simulink model "Dyn_6DoF_v2_0_r2019b"  (R2022a)
settings: Solver=ode4  StartTime=0.0  StopTime=simInit.TSIM  FixedStep=simInit.dt  MaxStep=simInit.dt  RelTol=1e-3
InitFcn:
  | close all
undefined symbols (not defined in the file): act, constr, DE2019, DiscIntNeverNeededParam, ENVMT, omega_rate_max, params, simInit
libraries: simulink x14, simulink_extras x3
(part 2 of 3)

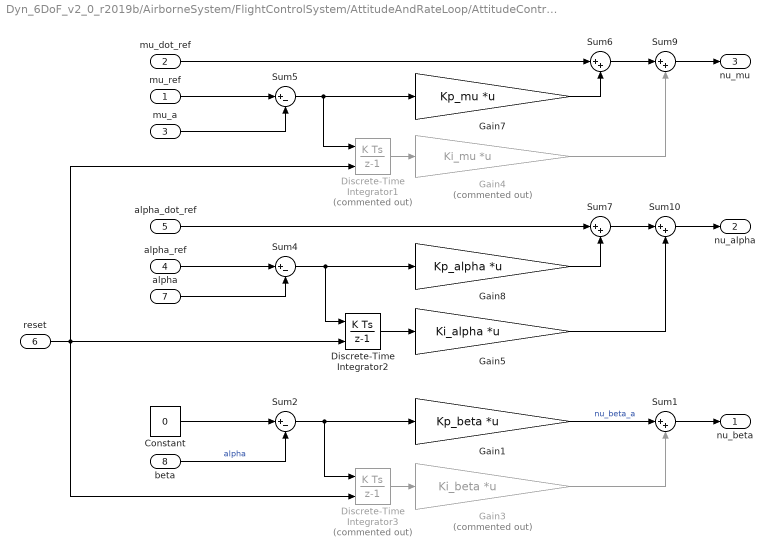
== system Dyn_6DoF_v2_0_r2019b/AirborneSystem/FlightControlSystem/AttitudeAndRateLoop/AttitudeController/PI-controller ==
  mu_ref : Inport
  mu_dot_ref : Inport  Port=2
  mu_a : Inport  Port=3
  alpha_ref : Inport  Port=4
  alpha_dot_ref : Inport  Port=5
  reset : Inport  Port=6
  alpha : Inport  Port=7
  beta : Inport  Port=8
  Constant : Constant  Value=0
  Discrete-Time Integrator1 : DiscreteIntegrator  Commented=on  ExternalReset=rising  SampleTime=-1  ICPrevOutput=DiscIntNeverNeededParam  ICPrevScaledInput=DiscIntNeverNeededParam
  Discrete-Time Integrator2 : DiscreteIntegrator  ExternalReset=either  SampleTime=-1  ICPrevOutput=DiscIntNeverNeededParam  ICPrevScaledInput=DiscIntNeverNeededParam
  Discrete-Time Integrator3 : DiscreteIntegrator  Commented=on  ExternalReset=rising  SampleTime=-1  ICPrevOutput=DiscIntNeverNeededParam  ICPrevScaledInput=DiscIntNeverNeededParam
  Gain1 : Gain  Gain=Kp_beta  Multiplication=Matrix(K*u)
  Gain3 : Gain  Commented=on  Gain=Ki_beta  Multiplication=Matrix(K*u)
  Gain4 : Gain  Commented=on  Gain=Ki_mu  Multiplication=Matrix(K*u)
  Gain5 : Gain  Gain=Ki_alpha  Multiplication=Matrix(K*u)
  Gain7 : Gain  Gain=Kp_mu  Multiplication=Matrix(K*u)
  Gain8 : Gain  Gain=Kp_alpha  Multiplication=Matrix(K*u)
  Sum{1,6..7,9..10} (5 alike) : Sum  Inputs=|++
  Sum2 : Sum  Inputs=|+-
  Sum4 : Sum  Inputs=|+-
  Sum5 : Sum  Inputs=|+-
  nu_beta : Outport  VectorParamsAs1DForOutWhenUnconnected=off
  nu_alpha : Outport  Port=2  VectorParamsAs1DForOutWhenUnconnected=off
  nu_mu : Outport  Port=3  VectorParamsAs1DForOutWhenUnconnected=off
  wires:
  Gain8/1 -> Sum7/2
  Gain5/1 -> Sum10/2
  Gain4/1 -> Sum9/2
  Sum7/1 -> Sum10/1
  Sum6/1 -> Sum9/1
  Gain7/1 -> Sum6/2
  Discrete-Time Integrator1/1 -> Gain4/1
  Sum4/1 -> Discrete-Time Integrator2/1, Gain8/1
  Sum5/1 -> Discrete-Time Integrator1/1, Gain7/1
  alpha/1 -> Sum4/2
  mu_a/1 -> Sum5/2
  alpha_ref/1 -> Sum4/1
  mu_ref/1 -> Sum5/1
  alpha_dot_ref/1 -> Sum7/1
  mu_dot_ref/1 -> Sum6/1
  reset/1 -> Discrete-Time Integrator2/2, Discrete-Time Integrator3/2, Discrete-Time Integrator1/2
  Constant/1 -> Sum2/1
  Sum2/1 -> Discrete-Time Integrator3/1, Gain1/1
  Gain1/1 -> Sum1/1  "nu_beta_a"
  beta/1 -> Sum2/2  "alpha"
  Gain3/1 -> Sum1/2
  Discrete-Time Integrator3/1 -> Gain3/1
  Sum1/1 -> nu_beta/1
  Sum10/1 -> nu_alpha/1
  Sum9/1 -> nu_mu/1
  Discrete-Time Integrator2/1 -> Gain5/1

== system Dyn_6DoF_v2_0_r2019b/AirborneSystem/FlightControlSystem/AttitudeAndRateLoop/AttitudeController/SecondOrderReferenceModel_alpha_a ==
  y_cmd : Inport
  hedge : Inport  Port=2
  Constant5 : Constant  Value=omega0_max
  Discrete-Time Integrator : DiscreteIntegrator  SampleTime=-1  LimitOutput=on  UpperSaturationLimit=y_max  LowerSaturationLimit=y_min  ICPrevOutput=DiscIntNeverNeededParam  ICPrevScaledInput=DiscIntNeverNeededParam
  Discrete-Time Integrator1 : DiscreteIntegrator  SampleTime=-1  LimitOutput=on  UpperSaturationLimit=yd_max  LowerSaturationLimit=yd_min  ICPrevOutput=DiscIntNeverNeededParam  ICPrevScaledInput=DiscIntNeverNeededParam
  Gain2 : Gain  Gain=2*zeta0
  Product : Product  Inputs=3
  Product1 : Product
  Saturation : Saturate  UpperLimit=y_max  LowerLimit=y_min
  Saturation1 : Saturate  UpperLimit=y2d_max  LowerLimit=y2d_min
  Sum : Sum  Inputs=|+-
  Sum1 : Sum  Inputs=|+-
  Sum2 : Sum  Inputs=|+-
  y_ref : Outport  VectorParamsAs1DForOutWhenUnconnected=off
  y_ref_dot : Outport  Port=2  VectorParamsAs1DForOutWhenUnconnected=off
  wires:
  Product/1 -> Sum/1
  Sum/1 -> Saturation1/1
  y_cmd/1 -> Saturation/1
  Saturation1/1 -> Discrete-Time Integrator1/1
  Gain2/1 -> Sum/2
  Sum1/1 -> Product/2
  Discrete-Time Integrator/1 -> Sum1/2, y_ref/1
  Discrete-Time Integrator1/1 -> y_ref_dot/1, Product1/1, Sum2/1
  Saturation/1 -> Sum1/1
  Sum2/1 -> Discrete-Time Integrator/1
  hedge/1 -> Sum2/2
  Product1/1 -> Gain2/1
  Constant5/1 -> Product1/2, Product/3, Product/1

== system Dyn_6DoF_v2_0_r2019b/AirborneSystem/FlightControlSystem/AttitudeAndRateLoop/AttitudeController/SecondOrderReferenceModel_mu_a ==
  y_cmd : Inport
  hedge : Inport  Port=2
  Constant5 : Constant  Value=omega0_max
  Discrete-Time Integrator : DiscreteIntegrator  SampleTime=-1  LimitOutput=on  UpperSaturationLimit=y_max  LowerSaturationLimit=y_min  ICPrevOutput=DiscIntNeverNeededParam  ICPrevScaledInput=DiscIntNeverNeededParam
  Discrete-Time Integrator1 : DiscreteIntegrator  SampleTime=-1  LimitOutput=on  UpperSaturationLimit=yd_max  LowerSaturationLimit=yd_min  ICPrevOutput=DiscIntNeverNeededParam  ICPrevScaledInput=DiscIntNeverNeededParam
  Gain2 : Gain  Gain=2*zeta0
  Product : Product  Inputs=3
  Product1 : Product
  Saturation : Saturate  UpperLimit=y_max  LowerLimit=y_min
  Saturation1 : Saturate  UpperLimit=y2d_max  LowerLimit=y2d_min
  Sum : Sum  Inputs=|+-
  Sum1 : Sum  Inputs=|+-
  Sum2 : Sum  Inputs=|+-
  y_ref : Outport  VectorParamsAs1DForOutWhenUnconnected=off
  y_ref_dot : Outport  Port=2  VectorParamsAs1DForOutWhenUnconnected=off
  wires:
  Discrete-Time Integrator/1 -> Sum1/2, y_ref/1
  Product/1 -> Sum/1
  y_cmd/1 -> Saturation/1
  Discrete-Time Integrator1/1 -> y_ref_dot/1, Product1/1, Sum2/1
  Sum/1 -> Saturation1/1
  Gain2/1 -> Sum/2
  Sum1/1 -> Product/2
  Saturation1/1 -> Discrete-Time Integrator1/1
  Saturation/1 -> Sum1/1
  Sum2/1 -> Discrete-Time Integrator/1
  hedge/1 -> Sum2/2
  Product1/1 -> Gain2/1
  Constant5/1 -> Product1/2, Product/3, Product/1

== system Dyn_6DoF_v2_0_r2019b/AirborneSystem/FlightControlSystem/AttitudeAndRateLoop/RateLoop/ControlAllocation ==
  deflections_actuator_output : Inport
  airdata : Inport  Port=2
  Delta_mom_cmd : Inport  Port=3
  Constant1 : Constant  Value=1e-6
  Gain14 : Gain  Gain=[1/ DE2019.b, 0, 0; 0, 1/ DE2019.c, 0; 0, 0, 1/ DE2019.b]  Multiplication=Matrix(K*u)
  Gain15 : Gain  Gain=DE2019.S_wing
  Gain3 : Gain  Gain=0.5*ENVMT.rhos
  Product : Product  Inputs=*/
  Product2 : Product
  Selector : Selector  InputPortWidth=3  IndexOptions=Index vector (dialog)  Indices=1  OutputSizes=1
  Selector1 : Selector  InputPortWidth=3  IndexOptions=Index vector (dialog)  Indices=2  OutputSizes=1
  Sum13 : Sum
  Sum2 : Sum  Inputs=|++
  allocation : MATLAB Function  TreatAsAtomicUnit=on
  deflections_cmd : Outport  VectorParamsAs1DForOutWhenUnconnected=off
  wires:
  Selector1/1 -> allocation/2(alpha)
  airdata/1 -> Selector/1, Selector1/1
  Product2/1 -> Gain3/1
  Selector/1 -> Product2/1, Product2/2
  deflections_actuator_output/1 -> Sum13/1
  Gain14/1 -> allocation/1(dC_pqr)
  Sum13/1 -> deflections_cmd/1
  allocation/1(Delta_deltas) -> Sum13/2
  Sum2/1 -> Product/2
  Constant1/1 -> Sum2/2
  Gain3/1 -> Gain15/1
  Gain15/1 -> Sum2/1
  Product/1 -> Gain14/1
  Delta_mom_cmd/1 -> Product/1

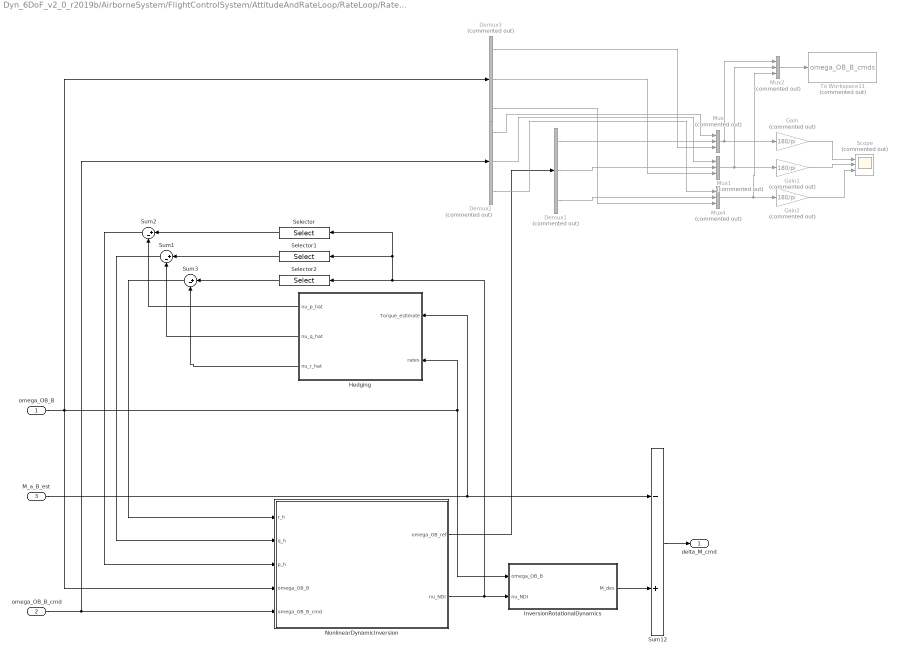
== system Dyn_6DoF_v2_0_r2019b/AirborneSystem/FlightControlSystem/AttitudeAndRateLoop/RateLoop/Rate_Loop ==
  omega_OB_B : Inport
  omega_OB_B_cmd : Inport  Port=2  PortDimensions=[3,1]
  M_a_B_est : Inport  Port=3  PortDimensions=[3,1]
  Demux1 : Demux  Commented=on  Outputs=3
  Demux2 : Demux  Commented=on  Outputs=3
  Demux3 : Demux  Commented=on  Outputs=3
  Gain : Gain  Commented=on  Gain=180/pi
  Gain1 : Gain  Commented=on  Gain=180/pi
  Gain2 : Gain  Commented=on  Gain=180/pi
  Hedging : Subsystem
  InversionRotationalDynamics : MATLAB Function  TreatAsAtomicUnit=on
  Mux{,1..2,4} (4 alike) : Mux  Commented=on  Inputs=3
  NonlinearDynamicInversion : Subsystem
  Scope : Scope  Commented=on  NumInputPorts=3
  Selector : Selector  InputPortWidth=3  IndexOptions=Index vector (dialog)  Indices=1  OutputSizes=1
  Selector1 : Selector  InputPortWidth=3  IndexOptions=Index vector (dialog)  Indices=2  OutputSizes=1
  Selector2 : Selector  InputPortWidth=3  IndexOptions=Index vector (dialog)  Indices=3  OutputSizes=1
  Sum1 : Sum  Inputs=|+-
  Sum12 : Sum  Inputs=-+
  Sum2 : Sum  Inputs=|+-
  Sum3 : Sum  Inputs=|+-
  To Workspace11 : ToWorkspace  Commented=on  VariableName=omega_OB_B_cmds  SaveFormat=Timeseries  SampleTime=-1
  delta_M_cmd : Outport  VectorParamsAs1DForOutWhenUnconnected=off
  wires:
  Mux2/1 -> To Workspace11/1
  omega_OB_B_cmd/1 -> Demux2/1, NonlinearDynamicInversion/5(omega_OB_B_cmd)
  Selector/1 -> Sum2/1
  Selector1/1 -> Sum1/1
  Selector2/1 -> Sum3/1
  NonlinearDynamicInversion/1(omega_OB_ref) -> Demux1/1
  Sum3/1 -> NonlinearDynamicInversion/1(r_h)
  Sum1/1 -> NonlinearDynamicInversion/2(q_h)
  Sum2/1 -> NonlinearDynamicInversion/3(p_h)
  Hedging/3(nu_r_hat) -> Sum3/2
  Hedging/2(nu_q_hat) -> Sum1/2
  Hedging/1(nu_p_hat) -> Sum2/2
  Sum12/1 -> delta_M_cmd/1
  InversionRotationalDynamics/1(M_des) -> Sum12/2
  M_a_B_est/1 -> Hedging/1(Torque_estimate), Sum12/1
  Gain1/1 -> Scope/2
  Mux/1 -> Gain/1, Mux2/1
  Mux1/1 -> Gain1/1, Mux2/2
  Demux1/1 -> Mux/2
  Demux1/2 -> Mux1/2
  Demux1/3 -> Mux4/2
  Mux4/1 -> Gain2/1, Mux2/3
  Gain2/1 -> Scope/3
  Gain/1 -> Scope/1
  Demux2/1 -> Mux/1
  Demux2/2 -> Mux1/1
  Demux2/3 -> Mux4/1
  Demux3/1 -> Mux/3
  Demux3/2 -> Mux1/3
  Demux3/3 -> Mux4/3
  omega_OB_B/1 -> Demux3/1, Hedging/2(rates), InversionRotationalDynamics/1(omega_OB_B), NonlinearDynamicInversion/4(omega_OB_B)
  NonlinearDynamicInversion/2(nu_NDI) -> Selector/1, Selector1/1, Selector2/1, InversionRotationalDynamics/2(nu_NDI)

== system Dyn_6DoF_v2_0_r2019b/AirborneSystem/ForcesAndTorques/aerodynamic forces FSI/Wing Aero/If Action Subsystem ==
  FSI_in : Inport
  simTime : Inport  Port=2
  Action Port : ActionPort  ActionPortLabel=if(u1 >= 1)
  Demux1 : Demux  Outputs=6
  FSI_sim : MATLABFcn  Commented=on  MATLABFcn=Init_FSIsim  OutputDimensions=[6,1]  Output1D=off
  MATLAB Function : MATLAB Function  TreatAsAtomicUnit=on
  Mux6 : Mux  Inputs=2
  Terminator{1..5,7} (6 alike) : Terminator  Commented=on
  FSI_out : Outport  VectorParamsAs1DForOutWhenUnconnected=off
  wires:
  Demux1/1 -> Terminator7/1  "Fx"
  Demux1/6 -> Terminator1/1  "Myaw"
  simTime/1 -> Mux6/2
  Mux6/1 -> MATLAB Function/1(u)
  Demux1/5 -> Terminator2/1  "Mpitch"
  Demux1/2 -> Terminator3/1  "Fy"
  FSI_in/1 -> Mux6/1
  MATLAB Function/1(y) -> FSI_out/1, Demux1/1
  Demux1/3 -> Terminator5/1  "Fz"
  Demux1/4 -> Terminator4/1  "Mroll"

== system Dyn_6DoF_v2_0_r2019b/AirborneSystem/ForcesAndTorques/aerodynamic forces FSI/Wing Aero/If Action Subsystem1 ==
  Simple_in : Inport
  Action Port : ActionPort  ActionPortLabel=else
  FSI : Subsystem
  Simple_out : Outport  VectorParamsAs1DForOutWhenUnconnected=off
  wires:
  Simple_in/1 -> FSI/1(In1)
  FSI/1(Out1) -> Simple_out/1

== system Dyn_6DoF_v2_0_r2019b/AirborneSystem/FlightControlSystem/AttitudeAndRateLoop/RateLoop/Rate_Loop/Hedging ==
  Torque_estimate : Inport
  rates : Inport  Port=2
  Demux1 : Demux  Outputs=3
  InversionRotationalDynamics1 : MATLAB Function  TreatAsAtomicUnit=on
  Signal Specification : SignalSpecification  Dimensions=[3,1]
  nu_p_hat : Outport  VectorParamsAs1DForOutWhenUnconnected=off
  nu_q_hat : Outport  Port=2  VectorParamsAs1DForOutWhenUnconnected=off
  nu_r_hat : Outport  Port=3  VectorParamsAs1DForOutWhenUnconnected=off
  wires:
  Signal Specification/1 -> InversionRotationalDynamics1/1(Moments)
  Torque_estimate/1 -> Signal Specification/1
  InversionRotationalDynamics1/3(nu_r_hat) -> nu_r_hat/1
  InversionRotationalDynamics1/2(nu_q_hat) -> nu_q_hat/1
  rates/1 -> Demux1/1
  InversionRotationalDynamics1/1(nu_p_hat) -> nu_p_hat/1
  Demux1/2 -> InversionRotationalDynamics1/3(q)
  Demux1/1 -> InversionRotationalDynamics1/2(p)
  Demux1/3 -> InversionRotationalDynamics1/4(r)

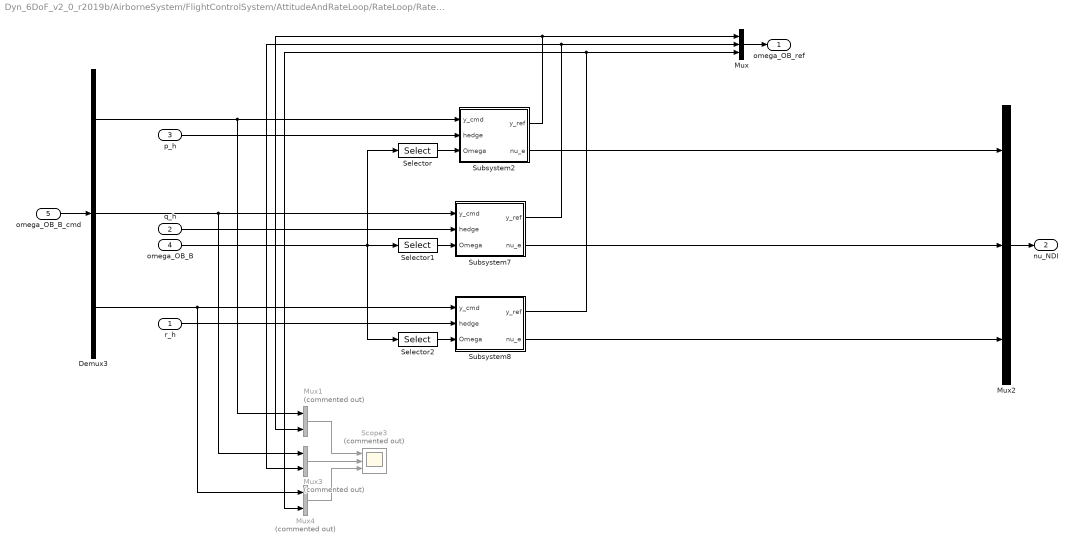
== system Dyn_6DoF_v2_0_r2019b/AirborneSystem/FlightControlSystem/AttitudeAndRateLoop/RateLoop/Rate_Loop/NonlinearDynamicInversion ==
  r_h : Inport
  q_h : Inport  Port=2
  p_h : Inport  Port=3
  omega_OB_B : Inport  Port=4
  omega_OB_B_cmd : Inport  Port=5
  Demux3 : Demux  Outputs=3
  Mux : Mux  Inputs=3
  Mux1 : Mux  Commented=on  Inputs=2
  Mux2 : Mux  Inputs=3
  Mux3 : Mux  Commented=on  Inputs=2
  Mux4 : Mux  Commented=on  Inputs=2
  Scope3 : Scope  Commented=on  NumInputPorts=3
  Selector : Selector  InputPortWidth=3  IndexOptions=Index vector (dialog)  Indices=1  OutputSizes=1
  Selector1 : Selector  InputPortWidth=3  IndexOptions=Index vector (dialog)  Indices=2  OutputSizes=1
  Selector2 : Selector  InputPortWidth=3  IndexOptions=Index vector (dialog)  Indices=3  OutputSizes=1
  Subsystem2 : Subsystem  mask{w0_max=params.w0_p_max, Kp=params.Kp_p, Ki=0}
      mask prompts: w0_max "omega0_max"
  Subsystem7 : Subsystem  mask{w0_max=params.w0_q_max, Kp=params.Kp_q, Ki=0}
      mask prompts: w0_max "omega0_max"
  Subsystem8 : Subsystem  mask{w0_max=params.w0_r_max, Kp=params.Kp_r, Ki=0}
      mask prompts: w0_max "omega0_max"
  omega_OB_ref : Outport  VectorParamsAs1DForOutWhenUnconnected=off
  nu_NDI : Outport  Port=2  VectorParamsAs1DForOutWhenUnconnected=off
  wires:
  omega_OB_B_cmd/1 -> Demux3/1
  Mux/1 -> omega_OB_ref/1
  Demux3/1 -> Subsystem2/1(y_cmd), Mux1/1
  omega_OB_B/1 -> Selector2/1, Selector1/1, Selector/1
  Demux3/2 -> Subsystem7/1(y_cmd), Mux3/1
  Demux3/3 -> Subsystem8/1(y_cmd), Mux4/1
  Mux2/1 -> nu_NDI/1
  Mux1/1 -> Scope3/1
  Mux3/1 -> Scope3/2
  Mux4/1 -> Scope3/3
  Subsystem2/1(y_ref) -> Mux1/2, Mux/1
  p_h/1 -> Subsystem2/2(hedge)
  Subsystem2/2(nu_e) -> Mux2/1
  Subsystem7/1(y_ref) -> Mux3/2, Mux/2
  q_h/1 -> Subsystem7/2(hedge)
  Subsystem7/2(nu_e) -> Mux2/2
  Subsystem8/1(y_ref) -> Mux4/2, Mux/3
  r_h/1 -> Subsystem8/2(hedge)
  Subsystem8/2(nu_e) -> Mux2/3
  Selector/1 -> Subsystem2/3(Omega)
  Selector1/1 -> Subsystem7/3(Omega)
  Selector2/1 -> Subsystem8/3(Omega)

== system Dyn_6DoF_v2_0_r2019b/AirborneSystem/ForcesAndTorques/aerodynamic forces FSI/Wing Aero/If Action Subsystem1/FSI ==
  In1 : Inport
  1-D Lookup Table : Lookup_n-D  NumberOfTableDimensions=1  BreakpointsForDimension1=DE2019.initAircraft.alpha  BreakpointsForDimension2=[1 1]  Table=DE2019.initAircraft.wing_cL_Static'  InternalRulePriority=Speed  RndMeth=Simplest
  1-D Lookup Table1 : Lookup_n-D  NumberOfTableDimensions=1  BreakpointsForDimension1=DE2019.initAircraft.alpha  BreakpointsForDimension2=[1 1]  Table=DE2019.initAircraft.wing_cD_Static'  InternalRulePriority=Speed  RndMeth=Simplest
  1-D Lookup Table4 : Lookup_n-D  NumberOfTableDimensions=1  BreakpointsForDimension1=DE2019.initAircraft.alpha  BreakpointsForDimension2=[1 1]  Table=DE2019.initAircraft.wing_cM_Static'  InternalRulePriority=Speed  RndMeth=Simplest
  Demux : Demux  Outputs=5
  Gain1 : Gain  Gain=DE2019.initAircraft.wing_cRoll_Static
  Mux6 : Mux  Inputs=6
  Radians to Degrees : simulink_extras/Transformations/Radians to Degrees
  Saturation : Saturate  UpperLimit=max(DE2019.initAircraft.alpha)  LowerLimit=min(DE2019.initAircraft.alpha)
  Saturation3 : Saturate  UpperLimit=act.aileron.max_deflection  LowerLimit=act.aileron.min_deflection
  Simple_wing_aero : MATLAB Function  TreatAsAtomicUnit=on
  Subsystem1 : Subsystem
  Sum3 : Sum  Inputs=+-
  Out1 : Outport  VectorParamsAs1DForOutWhenUnconnected=off
  wires:
  Simple_wing_aero/1(out) -> Out1/1
  In1/1 -> Demux/1
  Mux6/1 -> Simple_wing_aero/1(input)
  Saturation/1 -> 1-D Lookup Table4/1, 1-D Lookup Table1/1, 1-D Lookup Table/1
  Demux/2 -> Subsystem1/1(alpha), Radians to Degrees/1, Mux6/2
  1-D Lookup Table1/1 -> Mux6/4
  1-D Lookup Table/1 -> Mux6/3
  1-D Lookup Table4/1 -> Mux6/5
  Demux/3 -> Subsystem1/2(beta)
  Radians to Degrees/1 -> Saturation/1
  Demux/1 -> Subsystem1/3(velocity), Mux6/1
  Demux/4 -> Subsystem1/4(Omega)
  Demux/5 -> Sum3/1
  Subsystem1/1(defl_damp) -> Sum3/2
  Gain1/1 -> Mux6/6
  Sum3/1 -> Saturation3/1
  Saturation3/1 -> Gain1/1

== system Dyn_6DoF_v2_0_r2019b/AirborneSystem/FlightControlSystem/AttitudeAndRateLoop/RateLoop/Rate_Loop/NonlinearDynamicInversion/Subsystem2 ==
  y_cmd : Inport
  hedge : Inport  Port=2
  Omega : Inport  Port=3
  Roll_PI1 : Subsystem  mask{Kp=Kp, Ki=Ki}
      mask prompts: Kp "Kp_traction"; Ki "Ki_traction"
  SecondOrderReferenceModel_p : Subsystem  mask{omega0_max=w0_max, zeta0=1, y_max=constr.max_rates_B, y_min=-constr.max_rates_B, yd_max=inf, yd_min=-inf, y2d_max=inf, y2d_min=-inf}
  Sum : Sum
  y_ref : Outport
  nu_e : Outport  Port=2
  wires:
  Roll_PI1/1(nu_e) -> Sum/2
  SecondOrderReferenceModel_p/2(y_ref_dot) -> Sum/1
  y_cmd/1 -> SecondOrderReferenceModel_p/1(y_cmd)
  SecondOrderReferenceModel_p/1(y_ref) -> y_ref/1, Roll_PI1/1(p_ref)
  hedge/1 -> SecondOrderReferenceModel_p/2(hedge)
  Sum/1 -> nu_e/1
  Omega/1 -> Roll_PI1/2(p)

== system Dyn_6DoF_v2_0_r2019b/AirborneSystem/FlightControlSystem/AttitudeAndRateLoop/RateLoop/Rate_Loop/NonlinearDynamicInversion/Subsystem7 ==
  y_cmd : Inport
  hedge : Inport  Port=2
  Omega : Inport  Port=3
  Roll_PI1 : Subsystem  mask{Kp=Kp, Ki=Ki}
      mask prompts: Kp "Kp_traction"; Ki "Ki_traction"
  SecondOrderReferenceModel_p : Subsystem  mask{omega0_max=w0_max, zeta0=1, y_max=constr.max_rates_B, y_min=-constr.max_rates_B, yd_max=inf, yd_min=-inf, y2d_max=inf, y2d_min=-inf}
  Sum : Sum
  y_ref : Outport
  nu_e : Outport  Port=2
  wires:
  Roll_PI1/1(nu_e) -> Sum/2
  SecondOrderReferenceModel_p/2(y_ref_dot) -> Sum/1
  y_cmd/1 -> SecondOrderReferenceModel_p/1(y_cmd)
  SecondOrderReferenceModel_p/1(y_ref) -> y_ref/1, Roll_PI1/1(p_ref)
  hedge/1 -> SecondOrderReferenceModel_p/2(hedge)
  Sum/1 -> nu_e/1
  Omega/1 -> Roll_PI1/2(p)

== system Dyn_6DoF_v2_0_r2019b/AirborneSystem/FlightControlSystem/AttitudeAndRateLoop/RateLoop/Rate_Loop/NonlinearDynamicInversion/Subsystem8 ==
  y_cmd : Inport
  hedge : Inport  Port=2
  Omega : Inport  Port=3
  Roll_PI1 : Subsystem  mask{Kp=Kp, Ki=Ki}
      mask prompts: Kp "Kp_traction"; Ki "Ki_traction"
  SecondOrderReferenceModel_p : Subsystem  mask{omega0_max=w0_max, zeta0=1, y_max=constr.max_rates_B, y_min=-constr.max_rates_B, yd_max=inf, yd_min=-inf, y2d_max=inf, y2d_min=-inf}
  Sum : Sum
  y_ref : Outport
  nu_e : Outport  Port=2
  wires:
  Roll_PI1/1(nu_e) -> Sum/2
  SecondOrderReferenceModel_p/2(y_ref_dot) -> Sum/1
  y_cmd/1 -> SecondOrderReferenceModel_p/1(y_cmd)
  SecondOrderReferenceModel_p/1(y_ref) -> y_ref/1, Roll_PI1/1(p_ref)
  hedge/1 -> SecondOrderReferenceModel_p/2(hedge)
  Sum/1 -> nu_e/1
  Omega/1 -> Roll_PI1/2(p)

== system Dyn_6DoF_v2_0_r2019b/AirborneSystem/ForcesAndTorques/aerodynamic forces FSI/Wing Aero/If Action Subsystem1/FSI/Subsystem1 ==
  alpha : Inport
  beta : Inport  Port=2
  velocity : Inport  Port=3
  Omega : Inport  Port=4
  Atan2 : Trigonometry  Operator=atan2
  Constant : Constant  Value=(DE2019.b*0.75)
  Cos : Trigonometry  Operator=cos
  Cos1 : Trigonometry  Operator=cos
  Divide : Product  Inputs=*/
  Product : Product  Inputs=3
  Product3 : Product
  Selector : Selector  InputPortWidth=3  IndexOptions=Index vector (dialog)  Indices=1  OutputSizes=1
  max deflection (estimated) : Constant  Value=0.6109
  defl_damp : Outport  VectorParamsAs1DForOutWhenUnconnected=off
  wires:
  alpha/1 -> Cos/1
  beta/1 -> Cos1/1
  Product/1 -> Atan2/2
  velocity/1 -> Product/1
  Cos/1 -> Product/2
  Cos1/1 -> Product/3
  Constant/1 -> Product3/1
  Omega/1 -> Selector/1
  Selector/1 -> Product3/2
  Product3/1 -> Atan2/1
  Atan2/1 -> Divide/1
  max deflection (estimated)/1 -> Divide/2
  Divide/1 -> defl_damp/1

== system Dyn_6DoF_v2_0_r2019b/AirborneSystem/FlightControlSystem/AttitudeAndRateLoop/RateLoop/Rate_Loop/NonlinearDynamicInversion/Subsystem2/Roll_PI1 ==
  p_ref : Inport
  p : Inport  Port=2
  Constant1 : Constant  Value=Kp
  Constant3 : Constant  Value=Ki
  Discrete-Time Integrator1 : DiscreteIntegrator  SampleTime=-1  UpperSaturationLimit=omega_rate_max  LowerSaturationLimit=-omega_rate_max  ICPrevOutput=DiscIntNeverNeededParam  ICPrevScaledInput=DiscIntNeverNeededParam
  Product : Product
  Product2 : Product
  Sum : Sum  Inputs=|++
  Sum6 : Sum  Inputs=|+-
  nu_e : Outport  VectorParamsAs1DForOutWhenUnconnected=off
  wires:
  Sum/1 -> nu_e/1
  Discrete-Time Integrator1/1 -> Sum/2
  Sum6/1 -> Product2/1, Product/1
  Product2/1 -> Discrete-Time Integrator1/1
  p_ref/1 -> Sum6/1
  p/1 -> Sum6/2
  Product/1 -> Sum/1
  Constant1/1 -> Product/2
  Constant3/1 -> Product2/2

== system Dyn_6DoF_v2_0_r2019b/AirborneSystem/FlightControlSystem/AttitudeAndRateLoop/RateLoop/Rate_Loop/NonlinearDynamicInversion/Subsystem2/SecondOrderReferenceModel_p ==
  y_cmd : Inport
  hedge : Inport  Port=2
  Constant5 : Constant  Value=omega0_max
  Discrete-Time Integrator : DiscreteIntegrator  SampleTime=-1  LimitOutput=on  UpperSaturationLimit=y_max  LowerSaturationLimit=y_min  ICPrevOutput=DiscIntNeverNeededParam  ICPrevScaledInput=DiscIntNeverNeededParam
  Discrete-Time Integrator1 : DiscreteIntegrator  SampleTime=-1  LimitOutput=on  UpperSaturationLimit=yd_max  LowerSaturationLimit=yd_min  ICPrevOutput=DiscIntNeverNeededParam  ICPrevScaledInput=DiscIntNeverNeededParam
  Gain2 : Gain  Gain=2*zeta0
  Product : Product  Inputs=3
  Product1 : Product
  Saturation : Saturate  UpperLimit=y_max  LowerLimit=y_min
  Saturation1 : Saturate  UpperLimit=y2d_max  LowerLimit=y2d_min
  Sum : Sum  Inputs=|+-
  Sum1 : Sum  Inputs=|+-
  Sum2 : Sum  Inputs=|+-
  y_ref : Outport  VectorParamsAs1DForOutWhenUnconnected=off
  y_ref_dot : Outport  Port=2  VectorParamsAs1DForOutWhenUnconnected=off
  wires:
  Product/1 -> Sum/1
  Sum/1 -> Saturation1/1
  y_cmd/1 -> Saturation/1
  Saturation1/1 -> Discrete-Time Integrator1/1
  Gain2/1 -> Sum/2
  Sum1/1 -> Product/2
  Discrete-Time Integrator/1 -> Sum1/2, y_ref/1
  Discrete-Time Integrator1/1 -> y_ref_dot/1, Product1/1, Sum2/1
  Saturation/1 -> Sum1/1
  Sum2/1 -> Discrete-Time Integrator/1
  hedge/1 -> Sum2/2
  Product1/1 -> Gain2/1
  Constant5/1 -> Product1/2, Product/3, Product/1

== system Dyn_6DoF_v2_0_r2019b/AirborneSystem/FlightControlSystem/AttitudeAndRateLoop/RateLoop/Rate_Loop/NonlinearDynamicInversion/Subsystem7/Roll_PI1 ==
  p_ref : Inport
  p : Inport  Port=2
  Constant1 : Constant  Value=Kp
  Constant3 : Constant  Value=Ki
  Discrete-Time Integrator1 : DiscreteIntegrator  SampleTime=-1  UpperSaturationLimit=omega_rate_max  LowerSaturationLimit=-omega_rate_max  ICPrevOutput=DiscIntNeverNeededParam  ICPrevScaledInput=DiscIntNeverNeededParam
  Product : Product
  Product2 : Product
  Sum : Sum  Inputs=|++
  Sum6 : Sum  Inputs=|+-
  nu_e : Outport  VectorParamsAs1DForOutWhenUnconnected=off
  wires:
  Sum/1 -> nu_e/1
  Discrete-Time Integrator1/1 -> Sum/2
  Sum6/1 -> Product2/1, Product/1
  Product2/1 -> Discrete-Time Integrator1/1
  p_ref/1 -> Sum6/1
  p/1 -> Sum6/2
  Product/1 -> Sum/1
  Constant1/1 -> Product/2
  Constant3/1 -> Product2/2

== system Dyn_6DoF_v2_0_r2019b/AirborneSystem/FlightControlSystem/AttitudeAndRateLoop/RateLoop/Rate_Loop/NonlinearDynamicInversion/Subsystem7/SecondOrderReferenceModel_p ==
  y_cmd : Inport
  hedge : Inport  Port=2
  Constant5 : Constant  Value=omega0_max
  Discrete-Time Integrator : DiscreteIntegrator  SampleTime=-1  LimitOutput=on  UpperSaturationLimit=y_max  LowerSaturationLimit=y_min  ICPrevOutput=DiscIntNeverNeededParam  ICPrevScaledInput=DiscIntNeverNeededParam
  Discrete-Time Integrator1 : DiscreteIntegrator  SampleTime=-1  LimitOutput=on  UpperSaturationLimit=yd_max  LowerSaturationLimit=yd_min  ICPrevOutput=DiscIntNeverNeededParam  ICPrevScaledInput=DiscIntNeverNeededParam
  Gain2 : Gain  Gain=2*zeta0
  Product : Product  Inputs=3
  Product1 : Product
  Saturation : Saturate  UpperLimit=y_max  LowerLimit=y_min
  Saturation1 : Saturate  UpperLimit=y2d_max  LowerLimit=y2d_min
  Sum : Sum  Inputs=|+-
  Sum1 : Sum  Inputs=|+-
  Sum2 : Sum  Inputs=|+-
  y_ref : Outport  VectorParamsAs1DForOutWhenUnconnected=off
  y_ref_dot : Outport  Port=2  VectorParamsAs1DForOutWhenUnconnected=off
  wires:
  Product/1 -> Sum/1
  Sum/1 -> Saturation1/1
  y_cmd/1 -> Saturation/1
  Saturation1/1 -> Discrete-Time Integrator1/1
  Gain2/1 -> Sum/2
  Sum1/1 -> Product/2
  Discrete-Time Integrator/1 -> Sum1/2, y_ref/1
  Discrete-Time Integrator1/1 -> y_ref_dot/1, Product1/1, Sum2/1
  Saturation/1 -> Sum1/1
  Sum2/1 -> Discrete-Time Integrator/1
  hedge/1 -> Sum2/2
  Product1/1 -> Gain2/1
  Constant5/1 -> Product1/2, Product/3, Product/1

== system Dyn_6DoF_v2_0_r2019b/AirborneSystem/FlightControlSystem/AttitudeAndRateLoop/RateLoop/Rate_Loop/NonlinearDynamicInversion/Subsystem8/Roll_PI1 ==
  p_ref : Inport
  p : Inport  Port=2
  Constant1 : Constant  Value=Kp
  Constant3 : Constant  Value=Ki
  Discrete-Time Integrator1 : DiscreteIntegrator  SampleTime=-1  UpperSaturationLimit=omega_rate_max  LowerSaturationLimit=-omega_rate_max  ICPrevOutput=DiscIntNeverNeededParam  ICPrevScaledInput=DiscIntNeverNeededParam
  Product : Product
  Product2 : Product
  Sum : Sum  Inputs=|++
  Sum6 : Sum  Inputs=|+-
  nu_e : Outport  VectorParamsAs1DForOutWhenUnconnected=off
  wires:
  Sum/1 -> nu_e/1
  Discrete-Time Integrator1/1 -> Sum/2
  Sum6/1 -> Product2/1, Product/1
  Product2/1 -> Discrete-Time Integrator1/1
  p_ref/1 -> Sum6/1
  p/1 -> Sum6/2
  Product/1 -> Sum/1
  Constant1/1 -> Product/2
  Constant3/1 -> Product2/2

== system Dyn_6DoF_v2_0_r2019b/AirborneSystem/FlightControlSystem/AttitudeAndRateLoop/RateLoop/Rate_Loop/NonlinearDynamicInversion/Subsystem8/SecondOrderReferenceModel_p ==
  y_cmd : Inport
  hedge : Inport  Port=2
  Constant5 : Constant  Value=omega0_max
  Discrete-Time Integrator : DiscreteIntegrator  SampleTime=-1  LimitOutput=on  UpperSaturationLimit=y_max  LowerSaturationLimit=y_min  ICPrevOutput=DiscIntNeverNeededParam  ICPrevScaledInput=DiscIntNeverNeededParam
  Discrete-Time Integrator1 : DiscreteIntegrator  SampleTime=-1  LimitOutput=on  UpperSaturationLimit=yd_max  LowerSaturationLimit=yd_min  ICPrevOutput=DiscIntNeverNeededParam  ICPrevScaledInput=DiscIntNeverNeededParam
  Gain2 : Gain  Gain=2*zeta0
  Product : Product  Inputs=3
  Product1 : Product
  Saturation : Saturate  UpperLimit=y_max  LowerLimit=y_min
  Saturation1 : Saturate  UpperLimit=y2d_max  LowerLimit=y2d_min
  Sum : Sum  Inputs=|+-
  Sum1 : Sum  Inputs=|+-
  Sum2 : Sum  Inputs=|+-
  y_ref : Outport  VectorParamsAs1DForOutWhenUnconnected=off
  y_ref_dot : Outport  Port=2  VectorParamsAs1DForOutWhenUnconnected=off
  wires:
  Product/1 -> Sum/1
  Sum/1 -> Saturation1/1
  y_cmd/1 -> Saturation/1
  Saturation1/1 -> Discrete-Time Integrator1/1
  Gain2/1 -> Sum/2
  Sum1/1 -> Product/2
  Discrete-Time Integrator/1 -> Sum1/2, y_ref/1
  Discrete-Time Integrator1/1 -> y_ref_dot/1, Product1/1, Sum2/1
  Saturation/1 -> Sum1/1
  Sum2/1 -> Discrete-Time Integrator/1
  hedge/1 -> Sum2/2
  Product1/1 -> Gain2/1
  Constant5/1 -> Product1/2, Product/3, Product/1

== matlab function Dyn_6DoF_v2_0_r2019b/AirborneSystem/6DoFDynamics/Subsystem/MATLAB Function2 ==
  data: v_k_B input; DE2019 parameter; F_a_B input; F_p_B input; ENVMT parameter; F_t_W input; Torques_B input; vel_k_W input; omega_OB_B input; longlat input; EULER input; h_tau input; vel_K_B_dot output; M_OB output; omega_OB_B_dot output; longlat_dot output; eta_EULER_dot output; h_tau_dot output
% Copyright 2021 Delft University of Technology
%
% Licensed under the Apache License, Version 2.0 (the "License");
% you may not use this file except in compliance with the License.
% You may obtain a copy of the License at
%
%      http://www.apache.org/licenses/LICENSE-2.0
%
% Unless required by applicable law or agreed to in writing, software
% distributed under the License is distributed on an "AS IS" BASIS,
% WITHOUT WARRANTIES OR CONDITIONS OF ANY KIND, either express or implied.
% See the License for the specific language governing permissions and
% limitations under the License.

function [vel_K_B_dot, M_OB, omega_OB_B_dot, longlat_dot, ...
    eta_EULER_dot, h_tau_dot] = fcn(v_k_B, DE2019, F_a_B, F_p_B ,...
    ENVMT, F_t_W, Torques_B, vel_k_W, omega_OB_B, longlat, EULER, h_tau)
%fcn - 6DoF dynamics
%
% Inputs:
%    v_k_B      - Kinetic velocity in body reference frame
%    DE2019     - Aircraft parameters
%    F_a_B      - Aerodynamic forces acting on kite in body reference frame
%    F_p_B      - Propulsion and brake forces acting on kite in body
%                 reference frame
%    ENVMT      - Environment characteristics
%    F_t_W      - Tether force pulling at the kite
%    Torques_B  - Roll, pitch and yaw moments in body reference frame
%    vel_k_W    - Kinetic velocity in wind reference frame
%    omega_OB_B - Roll, pitch and yaw rates
%    longlat    - Longtitude, latitude
%    EULER      - Euler angles
%    h_tau      - Height in tau reference frame
%
% Outputs:
%    vel_K_B_dot    - Rate of change in kinetic velocity in body reference
%                     frame
%    M_OB           - Rotation matrix from body to inertial reference frame
%    omega_OB_B_dot - Roll, pitch and yaw accellerations
%    longlat_dot    - Rate of change of longtitude, latitude
%    eta_EULER_dot	- Rate of change of euler angles
%    h_tau_dot      - Rate of change of height in tau reference frame
%
%
% Author: Sebastian Rapp, Ph.D., Revised by: Dylan Eijkelhof, M.Sc.
% Delft University of Technology
% email address: d.eijkelhof@tudelft.nl
% December 2019; Last revision: 19-March-2021

%-------------	BEGIN CODE	--------------
% Preallocate variables
omega_OB_B_dot = zeros(3,1);
eta_EULER_dot  = zeros(3,1);
longlat_dot    = zeros(2,1);
vel_K_B_dot    = zeros(3,1);

c_psi = cos(EULER(3));
s_psi = sin(EULER(3));

c_theta = cos(EULER(2));
s_theta = sin(EULER(2));

c_phi = cos(EULER(1));
s_phi = sin(EULER(1)); 

M_OB = [ c_psi*c_theta, c_psi*s_theta*s_phi-s_psi*c_phi, c_psi*s_theta*c_phi+s_psi*s_phi;
         s_psi*c_theta, s_psi*s_theta*s_phi+c_psi*c_phi, s_psi*s_theta*c_phi-c_psi*s_phi;
        -s_theta, c_theta*s_phi, c_theta*c_phi];

long = longlat(1);
lat  = longlat(2);

F_g_O = [0;0;DE2019.mass*ENVMT.g];
F_t_O = transformFromOtoW( ENVMT.windDirection_rad, F_t_W);

%Forces to body fixed frame
F_g_t_B  = M_OB'*(F_g_O+F_t_O); 
Forces_B = F_a_B + F_g_t_B + F_p_B ;

p=omega_OB_B(1);
q=omega_OB_B(2);
r=omega_OB_B(3);

u=v_k_B(1);
v=v_k_B(2);
w=v_k_B(3);
vel_K_B_dot = [r*v-q*w + 1/DE2019.mass * Forces_B(1);
               p*w-r*u + 1/DE2019.mass * Forces_B(2);
               q*u-p*v + 1/DE2019.mass * Forces_B(3)];

c_theta = cos(EULER(2));
s_theta = sin(EULER(2));

c_phi = cos(EULER(1));
s_phi = sin(EULER(1)); 

eta_EULER_dot = [1 s_phi*s_theta/c_theta c_phi*s_theta/c_theta;
                 0 c_phi -s_phi; 
                 0 s_phi/c_theta c_phi/c_theta]*omega_OB_B;

Gamma  = DE2019.Jx*DE2019.Jz-DE2019.Jxz^2;
Gamma1 = (DE2019.Jxz*(DE2019.Jx - DE2019.Jy + DE2019.Jz ))/Gamma;
Gamma2 = (DE2019.Jz * (DE2019.Jz - DE2019.Jy) + DE2019.Jxz^2)/Gamma;
Gamma3 = DE2019.Jz/Gamma;
Gamma4 = DE2019.Jxz/Gamma;
Gamma5 = (DE2019.Jz - DE2019.Jx)/DE2019.Jy;
Gamma6 = DE2019.Jxz / DE2019.Jy;
Gamma7 = ((DE2019.Jx - DE2019.Jy)*DE2019.Jx + DE2019.Jxz^2 )/Gamma;
Gamma8 = DE2019.Jx / Gamma;

omega_OB_B_dot = [Gamma1 * p * q - Gamma2 * q * r + Gamma3 * Torques_B(1) + Gamma4 * Torques_B(3);
    Gamma5 * p * r - Gamma6 * (p^2 - r^2) + 1/DE2019.Jy *Torques_B(2);
     Gamma7 * p * q - Gamma1 * q * r + Gamma4 * Torques_B(1) + Gamma8 * Torques_B(3)];

%% Position propagation
sin_lat  = sin(lat);
sin_long = sin(long);
cos_lat  = cos(lat);
cos_long = cos(long);
 
M_tauW = [-sin_lat*cos_long, -sin_lat*sin_long,cos_lat;
    -sin_long, cos_long, 0;
    -cos_lat*cos_long, -cos_lat*sin_long, -sin_lat];

v_k_tau = M_tauW*vel_k_W;

long_dot = v_k_tau(2)/( abs(h_tau)*cos(lat));
lat_dot  = v_k_tau(1)/abs(h_tau);

h_tau_dot = -v_k_tau(3);

longlat_dot = [long_dot;
               lat_dot];

%-------------	END CODE	--------------
end

== matlab function Dyn_6DoF_v2_0_r2019b/AirborneSystem/FlightControlSystem/AttitudeAndRateLoop/AttitudeController/InversionAttitude ==
  data: omega_OB_B_cmd output size=[3,1]; mu_a input size=1; alpha input size=1; beta input size=1; nu_mu_a input size=1; nu_alpha_a input size=1; nu_beta_a input size=1; chi_a_dot_real input size=1; gamma_a_dot_real input size=1; gamma_a input; nu_hat output; constr parameter
% Copyright 2021 Delft University of Technology
%
% Licensed under the Apache License, Version 2.0 (the "License");
% you may not use this file except in compliance with the License.
% You may obtain a copy of the License at
%
%      http://www.apache.org/licenses/LICENSE-2.0
%
% Unless required by applicable law or agreed to in writing, software
% distributed under the License is distributed on an "AS IS" BASIS,
% WITHOUT WARRANTIES OR CONDITIONS OF ANY KIND, either express or implied.
% See the License for the specific language governing permissions and
% limitations under the License.

function [omega_OB_B_cmd, nu_hat]  = Attitude_inv( mu_a, alpha, beta, nu_mu_a,...
                                    nu_alpha_a, nu_beta_a, chi_a_dot_real,...
                                    gamma_a_dot_real, gamma_a, constr)
%Attitude_inv - Inverse attitude from error to actual
%
% Inputs:
%    mu_a               - Actual roll angle
%    alpha              - Actual pitch angle
%    beta               - Actual yaw angle
%    nu_mu_a            - Roll angle error w.r.t. actual with controller gains
%    nu_alpha_a         - Pitch angle error w.r.t. actual with controller gains
%    nu_beta_a          - Yaw angle error w.r.t. actual with controller gains
%    chi_a_dot_real     - Rate of change of course heading
%    gamma_a_dot_real   - Rate of change of path angle
%    gamma_a            - Actual aerodynamic path angle
%    constr             - Aircraft manoeuvre constraints
%
% Outputs:
%    omega_OB_B_cmd     - Commanded roll, pitch and yaw rates
%    nu_hat             - Expected error
%
%
% Author: Sebastian Rapp, Ph.D., Revised by: Dylan Eijkelhof, M.Sc.
% Delft University of Technology
% email address: d.eijkelhof@tudelft.nl
% December 2019; Last revision: 19-March-2021

%-------------	BEGIN CODE	--------------

c_m = cos(mu_a);
s_m = sin(mu_a);

c_a = cos(alpha);
s_a = sin(alpha);

c_b = cos(beta);
s_b = sin(beta);

M_B2ABar = zeros(3,3);

M_B2ABar(1,1) = c_a*c_b;
M_B2ABar(1,2) = s_b;
M_B2ABar(1,3) = s_a*c_b;
M_B2ABar(2,1) = -c_a*s_b*c_m+s_a*s_m;
M_B2ABar(2,2) = c_b*c_m;
M_B2ABar(2,3) = -s_a*s_b*c_m-s_m*c_a;
M_B2ABar(3,1) = -c_a*s_b*s_m-s_a*c_m;
M_B2ABar(3,2) = c_b*s_m;
M_B2ABar(3,3) = -s_a*s_b*s_m+c_a*c_m;


%% Inversion 

omega_OAbar_Abar = [-chi_a_dot_real*sin(gamma_a); 
                     gamma_a_dot_real; 
                     chi_a_dot_real*cos(gamma_a)];
                 
omega_OAbar_B = M_B2ABar'*omega_OAbar_Abar;
omega_OB_B_cmd =  [cos(alpha)*cos(beta) * nu_mu_a + nu_beta_a*sin(alpha); 
                  sin(beta)*nu_mu_a+nu_alpha_a;
                    sin(alpha)*cos(beta)*nu_mu_a - cos(alpha)*nu_beta_a] + omega_OAbar_B;

omega_OB_B_cmd_sat = max( min( omega_OB_B_cmd , constr.max_rates_B), -constr.max_rates_B ); 

% Expected pseudo-control
omega_AB_B = omega_OB_B_cmd_sat - M_B2ABar'*( [-chi_a_dot_real*sin(gamma_a);
                         gamma_a_dot_real; 
                         chi_a_dot_real*cos(gamma_a)]);
nu_x_hat = ( c_a*omega_AB_B(1) + s_a * omega_AB_B(3)  )/cos( beta );
nu_y_hat = -s_b*nu_x_hat  + omega_AB_B(2); 
nu_z_hat = ( omega_AB_B(1)*s_a - omega_AB_B(3) * c_a );
nu_hat = [nu_x_hat; nu_y_hat; nu_z_hat];

end

== matlab function Dyn_6DoF_v2_0_r2019b/AirborneSystem/FlightControlSystem/AttitudeAndRateLoop/RateLoop/ControlAllocation/allocation ==
  data: dC_pqr input; Delta_deltas output; alpha input; DE2019 parameter
% Copyright 2021 Delft University of Technology
%
% Licensed under the Apache License, Version 2.0 (the "License");
% you may not use this file except in compliance with the License.
% You may obtain a copy of the License at
%
%      http://www.apache.org/licenses/LICENSE-2.0
%
% Unless required by applicable law or agreed to in writing, software
% distributed under the License is distributed on an "AS IS" BASIS,
% WITHOUT WARRANTIES OR CONDITIONS OF ANY KIND, either express or implied.
% See the License for the specific language governing permissions and
% limitations under the License.

function Delta_deltas = fcn(dC_pqr, alpha, DE2019)
%Attitude_inv - Allocation matrix from moment increments to surface increments.
%
% Inputs:
%    dC_pqr        - Delta roll, pitch and yaw coefficients
%    alpha         - Actual pitch angle
%    DE2019        - Aircraft parameters
%
% Outputs:
%    Delta_deltas  - Delta actuator deflections
%
% Author: Sebastian Rapp, Ph.D., Revised by: Dylan Eijkelhof, M.Sc.
% Delft University of Technology
% email address: d.eijkelhof@tudelft.nl
% December 2019; Last revision: 19-March-2021

%-------------	BEGIN CODE	--------------
 
Cl_deltaA =DE2019.Cl_deltaA_0 + DE2019.Cl_deltaA_alpha * alpha + DE2019.Cl_deltaA_alpha2 * alpha^2;
Cl_deltaR =DE2019.Cl_deltaR_0 + DE2019.Cl_deltaR_alpha * alpha + DE2019.Cl_deltaR_alpha2 * alpha^2;                                 
 
Cm_deltaA =DE2019.Cm_deltaA_0 + DE2019.Cm_deltaA_alpha * alpha + DE2019.Cm_deltaA_alpha2 * alpha^2;  
Cm_deltaE = DE2019.Cm_deltaE_0  + DE2019.Cm_deltaE_alpha * alpha + DE2019.Cm_deltaE_alpha2 * alpha^2; 
 
Cn_deltaA =DE2019.Cn_deltaA_0 + DE2019.Cn_deltaA_alpha * alpha + DE2019.Cn_deltaA_alpha2 * alpha^2;  
Cn_deltaR =DE2019.Cn_deltaR_0 + DE2019.Cn_deltaR_alpha * alpha + DE2019.Cn_deltaR_alpha2 * alpha^2;
 
Ba = [[Cl_deltaA,0,Cl_deltaR];[Cm_deltaA,Cm_deltaE,0];[Cn_deltaA,0,Cn_deltaR]];
 
Delta_deltas = Ba\dC_pqr;

%-------------	END CODE	--------------
 
end

== matlab function Dyn_6DoF_v2_0_r2019b/AirborneSystem/ForcesAndTorques/aerodynamic forces FSI/Wing Aero/If Action Subsystem/MATLAB Function ==
  data: u input; y output
% Copyright 2021 Delft University of Technology
%
% Licensed under the Apache License, Version 2.0 (the "License");
% you may not use this file except in compliance with the License.
% You may obtain a copy of the License at
%
%      http://www.apache.org/licenses/LICENSE-2.0
%
% Unless required by applicable law or agreed to in writing, software
% distributed under the License is distributed on an "AS IS" BASIS,
% WITHOUT WARRANTIES OR CONDITIONS OF ANY KIND, either express or implied.
% See the License for the specific language governing permissions and
% limitations under the License.

function y = placeholder(u)

y = zeros(6,1);

== matlab function Dyn_6DoF_v2_0_r2019b/RequirementModelsAndLogging/MATLAB Function ==
  data: time input; eul input; stop_flag output; eul_old input
% Copyright 2021 Delft University of Technology
%
% Licensed under the Apache License, Version 2.0 (the "License");
% you may not use this file except in compliance with the License.
% You may obtain a copy of the License at
%
%      http://www.apache.org/licenses/LICENSE-2.0
%
% Unless required by applicable law or agreed to in writing, software
% distributed under the License is distributed on an "AS IS" BASIS,
% WITHOUT WARRANTIES OR CONDITIONS OF ANY KIND, either express or implied.
% See the License for the specific language governing permissions and
% limitations under the License.

function stop_flag = fcn(time, eul,eul_old)
phi = eul(1);
theta = eul(2);
% psi = eul(3);

phi_old = eul_old(1);
theta_old = eul_old(2);
% psi_old = eul_old(3);

if time>40
    if ((phi>pi/2 || phi<-pi/2) && sign(phi) ~= sign(phi_old))
        stop_flag = 1;
    elseif ((theta>pi/2 || theta<-pi/2) && sign(theta) ~= sign(theta_old))
        stop_flag = 1; 
%     elseif ((psi>pi/2 || psi<-pi/2) && sign(psi) ~= sign(psi_old))
%         stop_flag = 1; 
    else
        stop_flag = 0;
    end
else
    stop_flag = 0;
end
end

== matlab function Dyn_6DoF_v2_0_r2019b/RequirementModelsAndLogging/MATLAB Function1 ==
  data: Lift output; F_a_B input; Drag output; AoA input
% Copyright 2021 Delft University of Technology
%
% Licensed under the Apache License, Version 2.0 (the "License");
% you may not use this file except in compliance with the License.
% You may obtain a copy of the License at
%
%      http://www.apache.org/licenses/LICENSE-2.0
%
% Unless required by applicable law or agreed to in writing, software
% distributed under the License is distributed on an "AS IS" BASIS,
% WITHOUT WARRANTIES OR CONDITIONS OF ANY KIND, either express or implied.
% See the License for the specific language governing permissions and
% limitations under the License.

function [Lift, Drag]  = estimate_drag(F_a_B, AoA)
%estimate_drag - Transform drag from B to A reference frame
%
% Inputs:
%    F_a_B     - Aerodynamic forces in body reference frame
%    AoA       - Angle of Attack
%
% Outputs:
%    Drag    - Drag force
%
% Example: 
%    [Drag] = estimate_drag(F_a_B, AoA)
%
% Author: Sebastian Rapp, Ph.D., Revised by: Dylan Eijkelhof, M.Sc.
% Delft University of Technology
% email address: s.rapp@tudelft.nl
% email address: d.eijkelhof@tudelft.nl
% December 2019; Last revision: 06-October-2020

%-------------	BEGIN CODE	--------------

F_a_A = [cos(AoA), 0, sin(AoA);
    0, 1, 0; 
    -sin(AoA), 0, cos(AoA)] * F_a_B;

Lift = -F_a_A(3);
Drag = -F_a_A(1);

%-------------	 END CODE	--------------

end

== matlab function Dyn_6DoF_v2_0_r2019b/AirborneSystem/ForcesAndTorques/aerodynamic forces FSI/Wing Aero/If Action Subsystem1/FSI/Simple_wing_aero ==
  data: input input double; out output double size=[6,1]; DE2019 parameter; ENVMT parameter
% Copyright 2021 Delft University of Technology
%
% Licensed under the Apache License, Version 2.0 (the "License");
% you may not use this file except in compliance with the License.
% You may obtain a copy of the License at
%
%      http://www.apache.org/licenses/LICENSE-2.0
%
% Unless required by applicable law or agreed to in writing, software
% distributed under the License is distributed on an "AS IS" BASIS,
% WITHOUT WARRANTIES OR CONDITIONS OF ANY KIND, either express or implied.
% See the License for the specific language governing permissions and
% limitations under the License.

function out = simpleAero(input, DE2019, ENVMT)
%simpleAero - Main wing simple aero calculation
%
% Inputs:
%    input  - airspeed, AoA, CL, CD, CM and Croll
%    DE2019 - Aircraft parameters
%    ENVMT  - Environment characteristics
%
% Outputs:
%    out    - 3D forces and moments generated by the wing
%
%
% Author: Sebastian Rapp, Ph.D., Revised by: Dylan Eijkelhof, M.Sc.
% Delft University of Technology
% email address: d.eijkelhof@tudelft.nl
% December 2019; Last revision: 19-March-2021

%-------------	BEGIN CODE	--------------
    V = input(1);
    alpha = input(2);

    q = 0.5*ENVMT.rhos*V^2;

    F_L_main = -input(3)*q*DE2019.S_ref;
    F_D_main = input(4)*q*DE2019.S_ref;
    
    M_y_mw = input(5)*q*DE2019.S_wing*DE2019.c + ...
        (0.25*DE2019.c+DE2019.cog(1))*F_L_main;
    
    c_roll_mw = input(6);
    M_x_mw = (c_roll_mw) * q * DE2019.S_wing * DE2019.b;
    
    F_x_mw = -F_D_main*cos(alpha) - F_L_main*sin(alpha);
    F_z_mw = F_L_main*cos(alpha);


    out = [F_x_mw, 0, F_z_mw, M_x_mw, M_y_mw, 0]';
%-------------	END CODE	--------------
end

== matlab function Dyn_6DoF_v2_0_r2019b/AirborneSystem/6DoFDynamics/MATLAB Function3 ==
  data: v_w_O output; v_w_W input; ENVMT parameter
% Copyright 2021 Delft University of Technology
%
% Licensed under the Apache License, Version 2.0 (the "License");
% you may not use this file except in compliance with the License.
% You may obtain a copy of the License at
%
%      http://www.apache.org/licenses/LICENSE-2.0
%
% Unless required by applicable law or agreed to in writing, software
% distributed under the License is distributed on an "AS IS" BASIS,
% WITHOUT WARRANTIES OR CONDITIONS OF ANY KIND, either express or implied.
% See the License for the specific language governing permissions and
% limitations under the License.

function v_w_O = fcn(v_w_W, ENVMT)

v_w_O = transformFromWtoO(ENVMT.windDirection_rad, v_w_W );
end

== matlab function Dyn_6DoF_v2_0_r2019b/AirborneSystem/ForcesAndTorques/aerodynamic forces FSI/Elevator Aero/Elevator_aero ==
  data: input input double; out output double size=[6,1]; DE2019 parameter; ENVMT parameter
% Copyright 2021 Delft University of Technology
%
% Licensed under the Apache License, Version 2.0 (the "License");
% you may not use this file except in compliance with the License.
% You may obtain a copy of the License at
%
%      http://www.apache.org/licenses/LICENSE-2.0
%
% Unless required by applicable law or agreed to in writing, software
% distributed under the License is distributed on an "AS IS" BASIS,
% WITHOUT WARRANTIES OR CONDITIONS OF ANY KIND, either express or implied.
% See the License for the specific language governing permissions and
% limitations under the License.

function out = simpleAero(input, DE2019, ENVMT)
%simpleAero - Elevator simple aero calculation
%
% Inputs:
%    input  - airspeed, AoA, sideslip, CL and CD
%    DE2019 - Aircraft parameters
%    ENVMT  - Environment characteristics
%
% Outputs:
%    out    - 3D forces and moments generated by the elevator
%
%
% Author: Sebastian Rapp, Ph.D., Revised by: Dylan Eijkelhof, M.Sc.
% Delft University of Technology
% email address: d.eijkelhof@tudelft.nl
% December 2019; Last revision: 19-March-2021

%-------------	BEGIN CODE	--------------
    V = input(1);
    alpha = input(2);
    beta = input(3);

    q = 0.5*ENVMT.rhos*V^2;

    F_L_el = -input(4)*q*DE2019.S_el;
    F_D_el = -input(5)*q*DE2019.S_el;

    F_x_s = F_D_el*cos(alpha)*cos(beta) - F_L_el*sin(alpha)*cos(beta);
    F_y_s = 0;
    F_z_s = F_L_el*cos(alpha);

    M_x_s = 0;
    M_y_s = F_L_el*(DE2019.x_el+DE2019.c_el*0.25);
    M_z_s = 0;

    out = [F_x_s, F_y_s, F_z_s, M_x_s, M_y_s, M_z_s]';
%-------------	END CODE	--------------
end

== matlab function Dyn_6DoF_v2_0_r2019b/AirborneSystem/FlightControlSystem/AttitudeAndRateLoop/RateLoop/Rate_Loop/Hedging/InversionRotationalDynamics1 ==
  data: nu_p_hat output; Moments input; p input; q input; r input; DE2019 parameter; nu_q_hat output; nu_r_hat output
% Copyright 2021 Delft University of Technology
%
% Licensed under the Apache License, Version 2.0 (the "License");
% you may not use this file except in compliance with the License.
% You may obtain a copy of the License at
%
%      http://www.apache.org/licenses/LICENSE-2.0
%
% Unless required by applicable law or agreed to in writing, software
% distributed under the License is distributed on an "AS IS" BASIS,
% WITHOUT WARRANTIES OR CONDITIONS OF ANY KIND, either express or implied.
% See the License for the specific language governing permissions and
% limitations under the License.

function [nu_p_hat, nu_q_hat, nu_r_hat] = hedging_rot_inv(Moments, p, q, r, DE2019)
%hedging_rot_inv - Expected error after inversion
%
% Inputs:
%    Moments   - Roll, pitch and yaw moment
%    p         - Roll rate
%    q         - Pitch rate
%    r         - Yaw rate
%    DE2019    - Aircraft parameters
%
% Outputs:
%    nu_p_hat  - Expected roll rate error
%    nu_q_hat  - Expected pitch rate error
%    nu_r_hat  - Expected yaw rate error
%
% Other m-files required:   none
% Subfunctions:             none
% MAT-files required:       none
%
% Author: Sebastian Rapp, Ph.D., Revised by: Dylan Eijkelhof, M.Sc.
% Delft University of Technology
% email address: d.eijkelhof@tudelft.nl
% December 2019; Last revision: 19-March-2021

%------------- BEGIN CODE --------------
 
L = Moments(1); 
M = Moments(2); 
N = Moments(3); 

Jx =  DE2019.J(1,1); 
Jy =  DE2019.J(2,2); 
Jz =  DE2019.J(3,3); 
 
nu_p_hat = 1/Jx * (L - q * r * Jz +  q * r * Jy ); 
nu_q_hat = 1/Jy *(M - r * p * Jx + r * p * Jz  );
nu_r_hat = 1/Jz * (N - p * q * Jy + p * q * Jx ); 

%------------- END CODE --------------
end

== matlab function Dyn_6DoF_v2_0_r2019b/AirborneSystem/FlightControlSystem/AttitudeAndRateLoop/RateLoop/Rate_Loop/InversionRotationalDynamics ==
  data: omega_OB_B input; M_des output; nu_NDI input; DE2019 parameter
% Copyright 2021 Delft University of Technology
%
% Licensed under the Apache License, Version 2.0 (the "License");
% you may not use this file except in compliance with the License.
% You may obtain a copy of the License at
%
%      http://www.apache.org/licenses/LICENSE-2.0
%
% Unless required by applicable law or agreed to in writing, software
% distributed under the License is distributed on an "AS IS" BASIS,
% WITHOUT WARRANTIES OR CONDITIONS OF ANY KIND, either express or implied.
% See the License for the specific language governing permissions and
% limitations under the License.

function M_des  = Rate_inv(omega_OB_B,nu_NDI,  DE2019)
%Rate_inv - Determine desired moments
%
% Inputs:
%    omega_OB_B - Commanded roll, pitch and yaw rates
%    nu_NDI     - Roll, pitch and yaw rate error incl. controller gains
%    DE2019     - Aircraft parameters
%
% Outputs:
%    M_des  - Expected roll rate error
%
% Other m-files required:   none
% Subfunctions:             none
% MAT-files required:       none
%
% Author: Sebastian Rapp, Ph.D., Revised by: Dylan Eijkelhof, M.Sc.
% Delft University of Technology
% email address: d.eijkelhof@tudelft.nl
% December 2019; Last revision: 19-March-2021

%------------- BEGIN CODE --------------

p = omega_OB_B(1); 
q = omega_OB_B(2); 
r = omega_OB_B(3); 

nu_p = nu_NDI(1); 
nu_q = nu_NDI(2); 
nu_r = nu_NDI(3); 
 
Jx = DE2019.J(1,1); 
Jy = DE2019.J(2,2); 
Jz = DE2019.J(3,3);

Lc = Jx * nu_p + q * r * Jz  - q * r * Jy; 
Mc = Jy * nu_q + r * p * Jx - r * p * Jz;
Nc = Jz * nu_r + p * q * Jy - p * q * Jx; 

M_des = [Lc; Mc; Nc];

%------------- END CODE --------------
end
